simulink model "SimuModel_F_PDGravity"  (R2025b)
settings: Solver=ode45  StartTime=0.0  StopTime=t_d  MaxStep=Tc  RelTol=1e-8  AbsTol=1e-8
values from neighbouring files (symbols this model uses):
  F_e = K_r * k_t * inv(R_a) * k_v * K_r    [InitVariable_F.m]
  F_v = K_r * diag([0.01, 0.01]) * K_r    [InitVariable_F.m]
  g = 9.81    [InitVariable_F.m]
  G_r = K_r * k_t * inv(R_a) * G_v    [InitVariable_F.m]
  K_D = 75 * diag([1, 1])    [InitVariable_F.m]
  k_fp = k_tp    [InitVariable_F.m]
  K_P = 3750 * diag([1, 1])    [InitVariable_F.m]
  k_tp = K_r * k_tp    [InitVariable_F.m]
  k_tv = K_r * k_tv    [InitVariable_F.m]
  q_i = [-1.4706; 2.9413]    [InitVariable_F.m]
  Tc = 0.001    [InitVariable_F.m]
  Ts = Tc    (= 0.001)    [InitVariable_F.m]
undefined symbols (not defined in the file or in its folder): a, Ad, Bd, BMatrix, Cd, Dd, pi_l, pi_m
settings Model: ExtModeAutoUpdateStatusClock=off  Creator=luigivillani  LastModifiedBy=zj
settings SolverCC: AutoScaleAbsTol=off  InitialStep=0.1*Tc  AlgebraicLoopSolver=TrustRegion
settings DataIOCC: SaveFormat=Array  SignalLoggingSaveFormat=ModelDataLogs  SaveOutput=off  SaveTime=off  ReturnWorkspaceOutputs=off
settings OptimizationCC: BlockReduction=off  BooleanDataType=off  ExpressionDepthLimit=2147483647.0  InitFltsAndDblsToZero=on  LifeSpan=inf
settings DebuggingCC: SaveWithParameterizedLinksMsg=none  UnderspecifiedInitializationDetection=Classic  MergeDetectMultiDrivingBlocksExec=none  SignalResolutionControl=TryResolveAllWithWarning  MultiTaskDSMMsg=warning  MultiTaskCondExecSysMsg=none  FcnCallInpInsideContextMsg=warning  UnconnectedInputMsg=warning  UnconnectedOutputMsg=warning  UnconnectedLineMsg=warning  StateNameClashWarn=warning  SFUnexpectedBacktrackingDiag=warning  SFNoUnconditionalDefaultTransitionDiag=warning  SFExecutionAtInitializationDiag=none  ArithmeticOperatorsInVariantConditions=warning
settings HardwareCC: ProdBitPerPointer=32.0  ProdBitPerSizeT=32.0  ProdBitPerPtrDiffT=32.0  ProdLargestAtomicFloat=None  ProdIntDivRoundTo=Undefined  ProdEndianess=Unspecified  ProdWordSize=32.0  ProdHWDeviceType=32-bit Generic  TargetUnknown=on
settings ModelReferenceCC: EnableRefExpFcnMdlSchedulingChecks=on  PropagateSignalLabelsOutOfModel=off
settings SFSimCC: CustomCodeUndefinedFunction=UseInterfaceOnly
settings RTWCC: GPUComputeCapability=3.5
settings CodeAppCC: StateflowObjectComments=on
settings GRTTargetCC: TargetFcnLib=ansi_tfl_tmw.mat  TargetLangStandard=C89/C90 (ANSI)  CombineOutputUpdateFcns=off  GRTInterface=on
settings ConfigComp: CovMetricSettings=dw  CovSaveCumulativeToWorkspaceVar=on  CovSaveSingleToWorkspaceVar=on

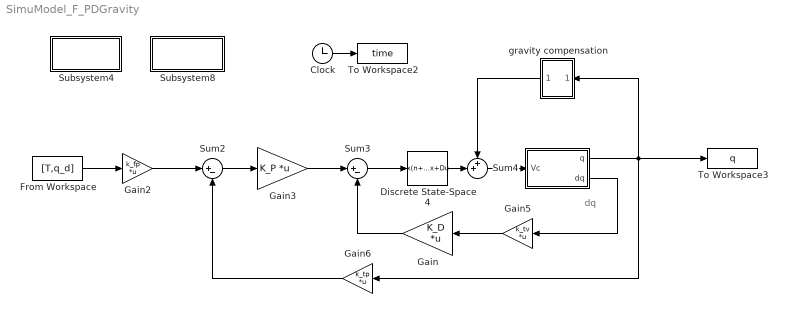
== system SimuModel_F_PDGravity ==
  note: dq
  " " : Subsystem
      mask Display: disp('Manipulator')
  Clock : Clock
  Discrete State-Space4 : DiscreteStateSpace  A=Ad  B=Bd  C=Cd  D=Dd  InitialCondition=[0 0]  SampleTime=Tc
      mask Display: disp('PI')
  From Workspace : FromWorkspace  VariableName=[T,q_d]  SampleTime=Tc  ZeroCross=off
  Gain : Gain  Gain=K_D  Multiplication=Matrix(K*u)
  Gain2 : Gain  Gain=k_fp  Multiplication=Matrix(K*u)  SampleTime=Tc
      mask Display: disp('k_fp')
  Gain3 : Gain  Gain=K_P  Multiplication=Matrix(K*u)  SampleTime=Tc
  Gain5 : Gain  Gain=k_tv  Multiplication=Matrix(K*u)  SampleTime=Tc
      mask Display: disp('k_tv')
  Gain6 : Gain  Gain=k_tp  Multiplication=Matrix(K*u)  SampleTime=Tc
      mask Display: disp('k_tp')
  Subsystem4 : Subsystem
      settings: OpenFcn=clear all;c=0;InitVariable_F;
      mask Display: disp('Init')
  Subsystem8 : Subsystem
      settings: OpenFcn=PlotFigure;
      mask Display: disp('plot')
  Sum2 : Sum  Inputs=|+-  InputSameDT=on  SaturateOnIntegerOverflow=on  OutDataTypeStr=Inherit: Same as first input
  Sum3 : Sum  Inputs=|+-  InputSameDT=on  SaturateOnIntegerOverflow=on  OutDataTypeStr=Inherit: Same as first input
  Sum4 : Sum  Inputs=++|  InputSameDT=on  SaturateOnIntegerOverflow=on  OutDataTypeStr=Inherit: Same as first input
  To Workspace2 : ToWorkspace  VariableName=time  SampleTime=Ts
      settings: MaxDataPoints=5001
  To Workspace3 : ToWorkspace  VariableName=q  SampleTime=Ts
      settings: MaxDataPoints=5001
  gravity compensation : Subsystem
      mask Display: disp('g(q)')
  wires:
  Sum2/1 -> Gain3/1
  Clock/1 -> To Workspace2/1
  " "/1(q) -> gravity compensation/1(in_1), Gain6/1, To Workspace3/1
  From Workspace/1 -> Gain2/1
  Gain2/1 -> Sum2/1
  " "/2(dq) -> Gain5/1
  Gain3/1 -> Sum3/1
  gravity compensation/1(out_1) -> Sum4/1
  Gain6/1 -> Sum2/2
  Gain/1 -> Sum3/2
  Gain5/1 -> Gain/1
  Sum3/1 -> Discrete State-Space4/1
  Sum4/1 -> " "/1(Vc)
  Discrete State-Space4/1 -> Sum4/2

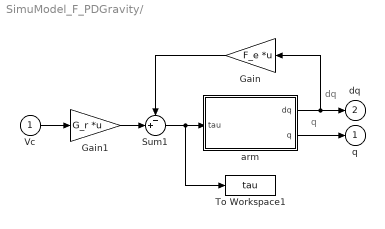
== system SimuModel_F_PDGravity/  ==
  note: dq
  note: q
  Vc : Inport
  Gain : Gain  Gain=F_e  Multiplication=Matrix(K*u)
  Gain1 : Gain  Gain=G_r  Multiplication=Matrix(K*u)
  Sum1 : Sum  Inputs=-+|  InputSameDT=on  SaturateOnIntegerOverflow=on  OutDataTypeStr=Inherit: Same as first input
  To Workspace1 : ToWorkspace  VariableName=tau  SampleTime=Ts
      settings: MaxDataPoints=5001
  arm : Subsystem
      mask Display: disp('inv(B(q))(tau-tau'')')
  q : Outport  InitialOutput=0  VectorParamsAs1DForOutWhenUnconnected=off
  dq : Outport  Port=2  InitialOutput=0  VectorParamsAs1DForOutWhenUnconnected=off
  wires:
  Vc/1 -> Gain1/1
  Gain1/1 -> Sum1/2
  Gain/1 -> Sum1/1
  arm/2("q ") -> q/1
  arm/1(dq) -> dq/1, Gain/1
  Sum1/1 -> To Workspace1/1, arm/1(tau)

== system SimuModel_F_PDGravity/Subsystem4 ==
  note: start

== system SimuModel_F_PDGravity/Subsystem8 ==
  note: start

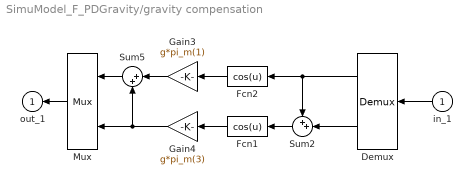
== system SimuModel_F_PDGravity/gravity compensation ==
  in_1 : Inport
  Demux : Demux  Outputs=2
      settings: DisplayOption=none
  Fcn1 : Fcn  Expr=cos(u)
  Fcn2 : Fcn  Expr=cos(u)
  Gain3 : Gain  Gain=g*pi_m(1)
  Gain4 : Gain  Gain=g*pi_m(3)
  Mux : Mux  Inputs=2
  Sum2 : Sum  Inputs=++|  InputSameDT=on  SaturateOnIntegerOverflow=on  OutDataTypeStr=Inherit: Same as first input
  Sum5 : Sum  Inputs=|++  InputSameDT=on  SaturateOnIntegerOverflow=on  OutDataTypeStr=Inherit: Same as first input
  out_1 : Outport  InitialOutput=0  VectorParamsAs1DForOutWhenUnconnected=off
  wires:
  in_1/1 -> Demux/1
  Demux/2 -> Sum2/2
  Sum2/1 -> Fcn1/1
  Fcn1/1 -> Gain4/1
  Fcn2/1 -> Gain3/1
  Demux/1 -> Fcn2/1, Sum2/1
  Gain3/1 -> Sum5/1
  Sum5/1 -> Mux/1
  Gain4/1 -> Sum5/2, Mux/2
  Mux/1 -> out_1/1

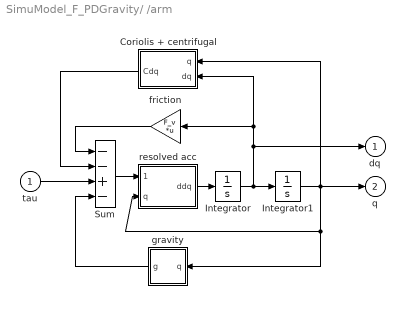
== system SimuModel_F_PDGravity/ /arm ==
  tau : Inport
  Coriolis + centrifugal : Subsystem
      mask Display: disp('C(q,dq)dq')
  Integrator : Integrator  InitialCondition=[0 0]  ZeroCross=off
  Integrator1 : Integrator  InitialCondition=q_i  ZeroCross=off
  Sum : Sum  Inputs=--+-  InputSameDT=on  SaturateOnIntegerOverflow=on  OutDataTypeStr=Inherit: Same as first input
  friction : Gain  Gain=F_v  Multiplication=Matrix(K*u)  SaturateOnIntegerOverflow=on  OutDataTypeStr=Inherit: Same as input  ParamDataTypeStr=Inherit: Same as input
      mask Display: disp('F_v')
  gravity : Subsystem
      mask Display: disp('g(q)')
  resolved acc : Subsystem
      mask Display: disp('inv(B(q))')
  dq : Outport  InitialOutput=0  VectorParamsAs1DForOutWhenUnconnected=off
  "q " : Outport  Port=2  InitialOutput=0  VectorParamsAs1DForOutWhenUnconnected=off
  wires:
  Coriolis + centrifugal/1(Cdq) -> Sum/2
  tau/1 -> Sum/3
  Integrator1/1 -> Coriolis + centrifugal/1(q), resolved acc/2(q), gravity/1(q), "q "/1
  resolved acc/1(ddq) -> Integrator/1
  Integrator/1 -> Integrator1/1, dq/1, Coriolis + centrifugal/2(dq), friction/1
  Sum/1 -> resolved acc/1(tau-tau')
  friction/1 -> Sum/1
  gravity/1(g) -> Sum/4

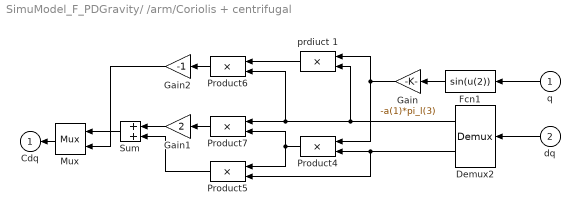
== system SimuModel_F_PDGravity/ /arm/Coriolis + centrifugal ==
  q : Inport
  dq : Inport  Port=2
  Demux2 : Demux  Outputs=2
      settings: DisplayOption=none
  Fcn1 : Fcn  Expr=sin(u(2))
  Gain : Gain  Gain=-a(1)*pi_l(3)  SaturateOnIntegerOverflow=on  OutDataTypeStr=Inherit: Same as input  ParamDataTypeStr=Inherit: Same as input
      mask Display: disp('k_3')
  Gain1 : Gain  Gain=2  SaturateOnIntegerOverflow=on  OutDataTypeStr=Inherit: Same as input  ParamDataTypeStr=Inherit: Same as input
  Gain2 : Gain  Gain=-1  SaturateOnIntegerOverflow=on  OutDataTypeStr=Inherit: Same as input  ParamDataTypeStr=Inherit: Same as input
  Mux : Mux  Inputs=2
  Product{4..7} (4 alike) : Product  InputSameDT=on  RndMeth=Zero  SaturateOnIntegerOverflow=on  OutDataTypeStr=Inherit: Same as first input
  Sum : Sum  InputSameDT=on  SaturateOnIntegerOverflow=on  OutDataTypeStr=Inherit: Same as first input
  prdiuct 1 : Product  InputSameDT=on  RndMeth=Zero  SaturateOnIntegerOverflow=on  OutDataTypeStr=Inherit: Same as first input
  Cdq : Outport  InitialOutput=0  VectorParamsAs1DForOutWhenUnconnected=off
  wires:
  dq/1 -> Demux2/1
  Gain2/1 -> Mux/2
  Product6/1 -> Gain2/1
  Mux/1 -> Cdq/1
  Sum/1 -> Mux/1
  Product5/1 -> Sum/2
  Gain1/1 -> Sum/1
  Product7/1 -> Gain1/1
  Demux2/1 -> prdiuct 1/2, Product6/2, Product7/1
  Demux2/2 -> Product4/2, Product5/2
  prdiuct 1/1 -> Product6/1
  Gain/1 -> prdiuct 1/1, Product4/1
  Fcn1/1 -> Gain/1
  q/1 -> Fcn1/1
  Product4/1 -> Product5/1, Product7/2

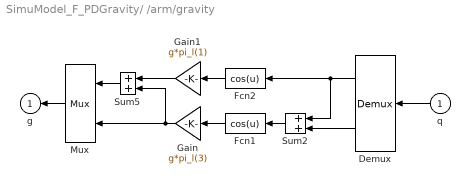
== system SimuModel_F_PDGravity/ /arm/gravity ==
  q : Inport
  Demux : Demux  Outputs=2
      settings: DisplayOption=none
  Fcn1 : Fcn  Expr=cos(u)
  Fcn2 : Fcn  Expr=cos(u)
  Gain : Gain  Gain=g*pi_l(3)  SaturateOnIntegerOverflow=on  OutDataTypeStr=Inherit: Same as input  ParamDataTypeStr=Inherit: Same as input
      mask Display: disp('k_2')
  Gain1 : Gain  Gain=g*pi_l(1)  SaturateOnIntegerOverflow=on  OutDataTypeStr=Inherit: Same as input  ParamDataTypeStr=Inherit: Same as input
      mask Display: disp('k_1')
  Mux : Mux  Inputs=2
  Sum2 : Sum  InputSameDT=on  SaturateOnIntegerOverflow=on  OutDataTypeStr=Inherit: Same as first input
  Sum5 : Sum  InputSameDT=on  SaturateOnIntegerOverflow=on  OutDataTypeStr=Inherit: Same as first input
  g : Outport  InitialOutput=0  VectorParamsAs1DForOutWhenUnconnected=off
  wires:
  q/1 -> Demux/1
  Demux/2 -> Sum2/2
  Sum2/1 -> Fcn1/1
  Fcn1/1 -> Gain/1
  Fcn2/1 -> Gain1/1
  Demux/1 -> Fcn2/1, Sum2/1
  Gain1/1 -> Sum5/1
  Sum5/1 -> Mux/1
  Gain/1 -> Sum5/2, Mux/2
  Mux/1 -> g/1

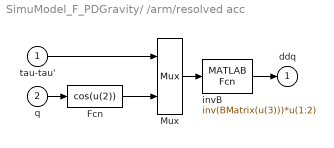
== system SimuModel_F_PDGravity/ /arm/resolved acc ==
  tau-tau' : Inport
  q : Inport  Port=2
  Fcn : Fcn  Expr=cos(u(2))
  Mux : Mux  Inputs=[2,1]
  "invB " : MATLABFcn  MATLABFcn=inv(BMatrix(u(3)))*u(1:2)  OutputDimensions=2
      mask Display: disp('inv(B(q))')
  ddq : Outport  InitialOutput=0  VectorParamsAs1DForOutWhenUnconnected=off
  wires:
  Fcn/1 -> Mux/2
  q/1 -> Fcn/1
  "invB "/1 -> ddq/1
  tau-tau'/1 -> Mux/1
  Mux/1 -> "invB "/1
